simulink model "rx2"  (R2022b)
settings: Solver=FixedStepDiscrete  StartTime=0.0  StopTime=3.3E6  FixedStep=1  RelTol=1e-3  EnableMultiTasking=on
model workspace (MAT data in the model file):
  mwTaskManagerKernelLatency = 0
undefined symbols (not defined in the file or in its folder): Add, jsin, magnitude, rom_pilot_conj_tt, Shift
libraries: hdlsllib x3231, whdlutilities x525, simulink x260, whdlmod x112, whdledac x26, dsphdlmathfun2 x24, commchan3 x1
(part 2 of 59)

== system rx2/process divide/transport_block3 ==
  data_in : Inport
  data_ctrl : Inport  Port=2  OutDataTypeStr=Bus: samplecontrol
  Bus Creator : BusCreator  Inputs=14
  Compare To Constant : hdlsllib/Logic and Bit Operations/Compare To Constant  relop===  const=1  OutDataTypeStr=boolean
  Compare To Constant1 : hdlsllib/Logic and Bit Operations/Compare To Constant  relop===  const=2  OutDataTypeStr=boolean
  Compare To Constant10 : hdlsllib/Logic and Bit Operations/Compare To Constant  relop===  const=11  OutDataTypeStr=boolean
  Compare To Constant11 : hdlsllib/Logic and Bit Operations/Compare To Constant  relop===  const=12  OutDataTypeStr=boolean
  Compare To Constant12 : hdlsllib/Logic and Bit Operations/Compare To Constant  relop===  const=13  OutDataTypeStr=boolean
  Compare To Constant13 : hdlsllib/Logic and Bit Operations/Compare To Constant  relop===  const=14  OutDataTypeStr=boolean
  Compare To Constant2 : hdlsllib/Logic and Bit Operations/Compare To Constant  relop===  const=3  OutDataTypeStr=boolean
  Compare To Constant3 : hdlsllib/Logic and Bit Operations/Compare To Constant  relop===  const=4  OutDataTypeStr=boolean
  Compare To Constant4 : hdlsllib/Logic and Bit Operations/Compare To Constant  relop===  const=5  OutDataTypeStr=boolean
  Compare To Constant5 : hdlsllib/Logic and Bit Operations/Compare To Constant  relop===  const=6  OutDataTypeStr=boolean
  Compare To Constant6 : hdlsllib/Logic and Bit Operations/Compare To Constant  relop===  const=7  OutDataTypeStr=boolean
  Compare To Constant7 : hdlsllib/Logic and Bit Operations/Compare To Constant  relop===  const=8  OutDataTypeStr=boolean
  Compare To Constant8 : hdlsllib/Logic and Bit Operations/Compare To Constant  relop===  const=9  OutDataTypeStr=boolean
  Compare To Constant9 : hdlsllib/Logic and Bit Operations/Compare To Constant  relop===  const=10  OutDataTypeStr=boolean
  Constant : Constant  Value=0  OutDataTypeStr=uint8
  Delay : Delay  DelayLength=1  InitialCondition=0
  Delay1 : Delay  DelayLength=1  InitialCondition=0
  HDL Counter : hdlsllib/Sources/HDL Counter  CountType=Count limited  CountInit=1  CountStep=1  CountMax=14  CountFromType=Initial value  CountFrom=1  CountResetPort=off  CountLoadPort=off  CountEnbPort=on  CountDirPort=off  CountHitOutputPort=off  CountDataType=Unsigned  CountWordLen=8  CountFracLen=0  CountSampTime=1
  Logical Operator : Logic  AllPortsSameDT=off  OutDataTypeStr=boolean
  Mux : Mux  Inputs=14
  Sample Control Bus Selector : whdlutilities/Sample Control Bus Selector  OutputSignals=start,end,valid
  Subsystem1 : Subsystem
  Subsystem10 : Subsystem
  Subsystem11 : Subsystem
  Subsystem12 : Subsystem
  Subsystem13 : Subsystem
  Subsystem14 : Subsystem
  Subsystem2 : Subsystem
  Subsystem3 : Subsystem
  Subsystem4 : Subsystem
  Subsystem5 : Subsystem
  Subsystem6 : Subsystem
  Subsystem7 : Subsystem
  Subsystem8 : Subsystem
  Subsystem9 : Subsystem
  Switch : Switch  Criteria=u2 ~= 0  SaturateOnIntegerOverflow=off  InputSameDT=off
  data_out : Outport  VectorParamsAs1DForOutWhenUnconnected=off
  valid_out : Outport  Port=2  OutDataTypeStr=Bus: RX_BUSOFDM1  VectorParamsAs1DForOutWhenUnconnected=off
  wires:
  data_in/1 -> Delay/1
  HDL Counter/1 -> Switch/1
  Compare To Constant/1 -> Subsystem1/2(select_valid)
  Compare To Constant1/1 -> Subsystem2/2(select_valid)
  Compare To Constant2/1 -> Subsystem3/2(select_valid)
  Compare To Constant3/1 -> Subsystem4/2(select_valid)
  Compare To Constant4/1 -> Subsystem5/2(select_valid)
  Compare To Constant5/1 -> Subsystem6/2(select_valid)
  Compare To Constant6/1 -> Subsystem7/2(select_valid)
  Compare To Constant7/1 -> Subsystem8/2(select_valid)
  Compare To Constant12/1 -> Subsystem13/2(select_valid)
  Compare To Constant11/1 -> Subsystem12/2(select_valid)
  Compare To Constant10/1 -> Subsystem11/2(select_valid)
  Compare To Constant9/1 -> Subsystem10/2(select_valid)
  Compare To Constant8/1 -> Subsystem9/2(select_valid)
  Delay1/1 -> Compare To Constant13/1, Compare To Constant12/1, Compare To Constant11/1, Compare To Constant10/1, Compare To Constant9/1, Compare To Constant8/1, Compare To Constant7/1, Compare To Constant6/1, Compare To Constant5/1, Compare To Constant4/1, Compare To Constant3/1, Compare To Constant2/1, Compare To Constant1/1, Compare To Constant/1
  Delay/1 -> Subsystem2/1(data_in), Subsystem3/1(data_in), Subsystem4/1(data_in), Subsystem5/1(data_in), Subsystem6/1(data_in), Subsystem7/1(data_in), Subsystem8/1(data_in), Subsystem9/1(data_in), Subsystem10/1(data_in), Subsystem11/1(data_in), Subsystem12/1(data_in), Subsystem14/1(data_in), Subsystem13/1(data_in), Subsystem1/1(data_in)
  Compare To Constant13/1 -> Subsystem14/2(select_valid)
  data_ctrl/1 -> Sample Control Bus Selector/1
  Sample Control Bus Selector/3 -> Logical Operator/2, Switch/2
  Switch/1 -> Delay1/1
  Constant/1 -> Switch/3
  Subsystem1/1(data_out) -> Mux/1
  Subsystem2/1(data_out) -> Mux/2
  Subsystem3/1(data_out) -> Mux/3
  Subsystem4/1(data_out) -> Mux/4
  Subsystem5/1(data_out) -> Mux/5
  Subsystem6/1(data_out) -> Mux/6
  Subsystem7/1(data_out) -> Mux/7
  Subsystem8/1(data_out) -> Mux/8
  Subsystem9/1(data_out) -> Mux/9
  Subsystem10/1(data_out) -> Mux/10
  Subsystem11/1(data_out) -> Mux/11
  Subsystem12/1(data_out) -> Mux/12
  Subsystem13/1(data_out) -> Mux/13
  Subsystem14/1(data_out) -> Mux/14
  Subsystem1/2(ctrl_out) -> Bus Creator/1
  Subsystem2/2(ctrl_out) -> Bus Creator/2
  Subsystem3/2(ctrl_out) -> Bus Creator/3
  Subsystem4/2(ctrl_out) -> Bus Creator/4
  Subsystem5/2(ctrl_out) -> Bus Creator/5
  Subsystem6/2(ctrl_out) -> Bus Creator/6
  Subsystem7/2(ctrl_out) -> Bus Creator/7
  Subsystem8/2(ctrl_out) -> Bus Creator/8
  Subsystem9/2(ctrl_out) -> Bus Creator/9
  Subsystem10/2(ctrl_out) -> Bus Creator/10
  Subsystem11/2(ctrl_out) -> Bus Creator/11
  Subsystem12/2(ctrl_out) -> Bus Creator/12
  Subsystem13/2(ctrl_out) -> Bus Creator/13
  Subsystem14/2(ctrl_out) -> Bus Creator/14
  Bus Creator/1 -> valid_out/1
  Mux/1 -> data_out/1
  Sample Control Bus Selector/2 -> Logical Operator/1
  Logical Operator/1 -> HDL Counter/1

== system rx2/process divide/transport_block4 ==
  data_in : Inport
  data_ctrl : Inport  Port=2  OutDataTypeStr=Bus: samplecontrol
  Bus Creator : BusCreator  Inputs=14
  Compare To Constant : hdlsllib/Logic and Bit Operations/Compare To Constant  relop===  const=1  OutDataTypeStr=boolean
  Compare To Constant1 : hdlsllib/Logic and Bit Operations/Compare To Constant  relop===  const=2  OutDataTypeStr=boolean
  Compare To Constant10 : hdlsllib/Logic and Bit Operations/Compare To Constant  relop===  const=11  OutDataTypeStr=boolean
  Compare To Constant11 : hdlsllib/Logic and Bit Operations/Compare To Constant  relop===  const=12  OutDataTypeStr=boolean
  Compare To Constant12 : hdlsllib/Logic and Bit Operations/Compare To Constant  relop===  const=13  OutDataTypeStr=boolean
  Compare To Constant13 : hdlsllib/Logic and Bit Operations/Compare To Constant  relop===  const=14  OutDataTypeStr=boolean
  Compare To Constant2 : hdlsllib/Logic and Bit Operations/Compare To Constant  relop===  const=3  OutDataTypeStr=boolean
  Compare To Constant3 : hdlsllib/Logic and Bit Operations/Compare To Constant  relop===  const=4  OutDataTypeStr=boolean
  Compare To Constant4 : hdlsllib/Logic and Bit Operations/Compare To Constant  relop===  const=5  OutDataTypeStr=boolean
  Compare To Constant5 : hdlsllib/Logic and Bit Operations/Compare To Constant  relop===  const=6  OutDataTypeStr=boolean
  Compare To Constant6 : hdlsllib/Logic and Bit Operations/Compare To Constant  relop===  const=7  OutDataTypeStr=boolean
  Compare To Constant7 : hdlsllib/Logic and Bit Operations/Compare To Constant  relop===  const=8  OutDataTypeStr=boolean
  Compare To Constant8 : hdlsllib/Logic and Bit Operations/Compare To Constant  relop===  const=9  OutDataTypeStr=boolean
  Compare To Constant9 : hdlsllib/Logic and Bit Operations/Compare To Constant  relop===  const=10  OutDataTypeStr=boolean
  Constant : Constant  Value=0  OutDataTypeStr=uint8
  Delay : Delay  DelayLength=1  InitialCondition=0
  Delay1 : Delay  DelayLength=1  InitialCondition=0
  HDL Counter : hdlsllib/Sources/HDL Counter  CountType=Count limited  CountInit=1  CountStep=1  CountMax=14  CountFromType=Initial value  CountFrom=1  CountResetPort=off  CountLoadPort=off  CountEnbPort=on  CountDirPort=off  CountHitOutputPort=off  CountDataType=Unsigned  CountWordLen=8  CountFracLen=0  CountSampTime=1
  Logical Operator : Logic  AllPortsSameDT=off  OutDataTypeStr=boolean
  Mux : Mux  Inputs=14
  Sample Control Bus Selector : whdlutilities/Sample Control Bus Selector  OutputSignals=start,end,valid
  Subsystem1 : Subsystem
  Subsystem10 : Subsystem
  Subsystem11 : Subsystem
  Subsystem12 : Subsystem
  Subsystem13 : Subsystem
  Subsystem14 : Subsystem
  Subsystem2 : Subsystem
  Subsystem3 : Subsystem
  Subsystem4 : Subsystem
  Subsystem5 : Subsystem
  Subsystem6 : Subsystem
  Subsystem7 : Subsystem
  Subsystem8 : Subsystem
  Subsystem9 : Subsystem
  Switch : Switch  Criteria=u2 ~= 0  SaturateOnIntegerOverflow=off  InputSameDT=off
  data_out : Outport  VectorParamsAs1DForOutWhenUnconnected=off
  valid_out : Outport  Port=2  OutDataTypeStr=Bus: RX_BUSOFDM1  VectorParamsAs1DForOutWhenUnconnected=off
  wires:
  Logical Operator/1 -> HDL Counter/1
  Sample Control Bus Selector/2 -> Logical Operator/1
  Mux/1 -> data_out/1
  Bus Creator/1 -> valid_out/1
  Subsystem14/2(ctrl_out) -> Bus Creator/14
  Subsystem13/2(ctrl_out) -> Bus Creator/13
  Subsystem12/2(ctrl_out) -> Bus Creator/12
  Subsystem11/2(ctrl_out) -> Bus Creator/11
  Subsystem10/2(ctrl_out) -> Bus Creator/10
  Subsystem9/2(ctrl_out) -> Bus Creator/9
  Subsystem8/2(ctrl_out) -> Bus Creator/8
  Subsystem7/2(ctrl_out) -> Bus Creator/7
  Subsystem6/2(ctrl_out) -> Bus Creator/6
  Subsystem5/2(ctrl_out) -> Bus Creator/5
  Subsystem4/2(ctrl_out) -> Bus Creator/4
  Subsystem3/2(ctrl_out) -> Bus Creator/3
  Subsystem2/2(ctrl_out) -> Bus Creator/2
  Subsystem1/2(ctrl_out) -> Bus Creator/1
  Subsystem14/1(data_out) -> Mux/14
  Subsystem13/1(data_out) -> Mux/13
  Subsystem12/1(data_out) -> Mux/12
  Subsystem11/1(data_out) -> Mux/11
  Subsystem10/1(data_out) -> Mux/10
  Subsystem9/1(data_out) -> Mux/9
  Subsystem8/1(data_out) -> Mux/8
  Subsystem7/1(data_out) -> Mux/7
  Subsystem6/1(data_out) -> Mux/6
  Subsystem5/1(data_out) -> Mux/5
  Subsystem4/1(data_out) -> Mux/4
  Subsystem3/1(data_out) -> Mux/3
  Subsystem2/1(data_out) -> Mux/2
  Subsystem1/1(data_out) -> Mux/1
  Constant/1 -> Switch/3
  Switch/1 -> Delay1/1
  Sample Control Bus Selector/3 -> Switch/2, Logical Operator/2
  data_ctrl/1 -> Sample Control Bus Selector/1
  Compare To Constant13/1 -> Subsystem14/2(select_valid)
  Delay/1 -> Subsystem1/1(data_in), Subsystem13/1(data_in), Subsystem14/1(data_in), Subsystem12/1(data_in), Subsystem11/1(data_in), Subsystem10/1(data_in), Subsystem9/1(data_in), Subsystem8/1(data_in), Subsystem7/1(data_in), Subsystem6/1(data_in), Subsystem5/1(data_in), Subsystem4/1(data_in), Subsystem3/1(data_in), Subsystem2/1(data_in)
  Delay1/1 -> Compare To Constant/1, Compare To Constant1/1, Compare To Constant2/1, Compare To Constant3/1, Compare To Constant4/1, Compare To Constant5/1, Compare To Constant6/1, Compare To Constant7/1, Compare To Constant8/1, Compare To Constant9/1, Compare To Constant10/1, Compare To Constant11/1, Compare To Constant12/1, Compare To Constant13/1
  Compare To Constant8/1 -> Subsystem9/2(select_valid)
  Compare To Constant9/1 -> Subsystem10/2(select_valid)
  Compare To Constant10/1 -> Subsystem11/2(select_valid)
  Compare To Constant11/1 -> Subsystem12/2(select_valid)
  Compare To Constant12/1 -> Subsystem13/2(select_valid)
  Compare To Constant7/1 -> Subsystem8/2(select_valid)
  Compare To Constant6/1 -> Subsystem7/2(select_valid)
  Compare To Constant5/1 -> Subsystem6/2(select_valid)
  Compare To Constant4/1 -> Subsystem5/2(select_valid)
  Compare To Constant3/1 -> Subsystem4/2(select_valid)
  Compare To Constant2/1 -> Subsystem3/2(select_valid)
  Compare To Constant1/1 -> Subsystem2/2(select_valid)
  Compare To Constant/1 -> Subsystem1/2(select_valid)
  HDL Counter/1 -> Switch/1
  data_in/1 -> Delay/1

== system rx2/process divide/transport_block5 ==
  data_in : Inport
  data_ctrl : Inport  Port=2  OutDataTypeStr=Bus: samplecontrol
  Bus Creator : BusCreator  Inputs=14
  Compare To Constant : hdlsllib/Logic and Bit Operations/Compare To Constant  relop===  const=1  OutDataTypeStr=boolean
  Compare To Constant1 : hdlsllib/Logic and Bit Operations/Compare To Constant  relop===  const=2  OutDataTypeStr=boolean
  Compare To Constant10 : hdlsllib/Logic and Bit Operations/Compare To Constant  relop===  const=11  OutDataTypeStr=boolean
  Compare To Constant11 : hdlsllib/Logic and Bit Operations/Compare To Constant  relop===  const=12  OutDataTypeStr=boolean
  Compare To Constant12 : hdlsllib/Logic and Bit Operations/Compare To Constant  relop===  const=13  OutDataTypeStr=boolean
  Compare To Constant13 : hdlsllib/Logic and Bit Operations/Compare To Constant  relop===  const=14  OutDataTypeStr=boolean
  Compare To Constant2 : hdlsllib/Logic and Bit Operations/Compare To Constant  relop===  const=3  OutDataTypeStr=boolean
  Compare To Constant3 : hdlsllib/Logic and Bit Operations/Compare To Constant  relop===  const=4  OutDataTypeStr=boolean
  Compare To Constant4 : hdlsllib/Logic and Bit Operations/Compare To Constant  relop===  const=5  OutDataTypeStr=boolean
  Compare To Constant5 : hdlsllib/Logic and Bit Operations/Compare To Constant  relop===  const=6  OutDataTypeStr=boolean
  Compare To Constant6 : hdlsllib/Logic and Bit Operations/Compare To Constant  relop===  const=7  OutDataTypeStr=boolean
  Compare To Constant7 : hdlsllib/Logic and Bit Operations/Compare To Constant  relop===  const=8  OutDataTypeStr=boolean
  Compare To Constant8 : hdlsllib/Logic and Bit Operations/Compare To Constant  relop===  const=9  OutDataTypeStr=boolean
  Compare To Constant9 : hdlsllib/Logic and Bit Operations/Compare To Constant  relop===  const=10  OutDataTypeStr=boolean
  Constant : Constant  Value=0  OutDataTypeStr=uint8
  Delay : Delay  DelayLength=1  InitialCondition=0
  Delay1 : Delay  DelayLength=1  InitialCondition=0
  HDL Counter : hdlsllib/Sources/HDL Counter  CountType=Count limited  CountInit=1  CountStep=1  CountMax=14  CountFromType=Initial value  CountFrom=1  CountResetPort=off  CountLoadPort=off  CountEnbPort=on  CountDirPort=off  CountHitOutputPort=off  CountDataType=Unsigned  CountWordLen=8  CountFracLen=0  CountSampTime=1
  Logical Operator : Logic  AllPortsSameDT=off  OutDataTypeStr=boolean
  Mux : Mux  Inputs=14
  Sample Control Bus Selector : whdlutilities/Sample Control Bus Selector  OutputSignals=start,end,valid
  Subsystem1 : Subsystem
  Subsystem10 : Subsystem
  Subsystem11 : Subsystem
  Subsystem12 : Subsystem
  Subsystem13 : Subsystem
  Subsystem14 : Subsystem
  Subsystem2 : Subsystem
  Subsystem3 : Subsystem
  Subsystem4 : Subsystem
  Subsystem5 : Subsystem
  Subsystem6 : Subsystem
  Subsystem7 : Subsystem
  Subsystem8 : Subsystem
  Subsystem9 : Subsystem
  Switch : Switch  Criteria=u2 ~= 0  SaturateOnIntegerOverflow=off  InputSameDT=off
  data_out : Outport  VectorParamsAs1DForOutWhenUnconnected=off
  valid_out : Outport  Port=2  OutDataTypeStr=Bus: RX_BUSOFDM1  VectorParamsAs1DForOutWhenUnconnected=off
  wires:
  data_in/1 -> Delay/1
  HDL Counter/1 -> Switch/1
  Compare To Constant/1 -> Subsystem1/2(select_valid)
  Compare To Constant1/1 -> Subsystem2/2(select_valid)
  Compare To Constant2/1 -> Subsystem3/2(select_valid)
  Compare To Constant3/1 -> Subsystem4/2(select_valid)
  Compare To Constant4/1 -> Subsystem5/2(select_valid)
  Compare To Constant5/1 -> Subsystem6/2(select_valid)
  Compare To Constant6/1 -> Subsystem7/2(select_valid)
  Compare To Constant7/1 -> Subsystem8/2(select_valid)
  Compare To Constant12/1 -> Subsystem13/2(select_valid)
  Compare To Constant11/1 -> Subsystem12/2(select_valid)
  Compare To Constant10/1 -> Subsystem11/2(select_valid)
  Compare To Constant9/1 -> Subsystem10/2(select_valid)
  Compare To Constant8/1 -> Subsystem9/2(select_valid)
  Delay1/1 -> Compare To Constant13/1, Compare To Constant12/1, Compare To Constant11/1, Compare To Constant10/1, Compare To Constant9/1, Compare To Constant8/1, Compare To Constant7/1, Compare To Constant6/1, Compare To Constant5/1, Compare To Constant4/1, Compare To Constant3/1, Compare To Constant2/1, Compare To Constant1/1, Compare To Constant/1
  Delay/1 -> Subsystem2/1(data_in), Subsystem3/1(data_in), Subsystem4/1(data_in), Subsystem5/1(data_in), Subsystem6/1(data_in), Subsystem7/1(data_in), Subsystem8/1(data_in), Subsystem9/1(data_in), Subsystem10/1(data_in), Subsystem11/1(data_in), Subsystem12/1(data_in), Subsystem14/1(data_in), Subsystem13/1(data_in), Subsystem1/1(data_in)
  Compare To Constant13/1 -> Subsystem14/2(select_valid)
  data_ctrl/1 -> Sample Control Bus Selector/1
  Sample Control Bus Selector/3 -> Logical Operator/2, Switch/2
  Switch/1 -> Delay1/1
  Constant/1 -> Switch/3
  Subsystem1/1(data_out) -> Mux/1
  Subsystem2/1(data_out) -> Mux/2
  Subsystem3/1(data_out) -> Mux/3
  Subsystem4/1(data_out) -> Mux/4
  Subsystem5/1(data_out) -> Mux/5
  Subsystem6/1(data_out) -> Mux/6
  Subsystem7/1(data_out) -> Mux/7
  Subsystem8/1(data_out) -> Mux/8
  Subsystem9/1(data_out) -> Mux/9
  Subsystem10/1(data_out) -> Mux/10
  Subsystem11/1(data_out) -> Mux/11
  Subsystem12/1(data_out) -> Mux/12
  Subsystem13/1(data_out) -> Mux/13
  Subsystem14/1(data_out) -> Mux/14
  Subsystem1/2(ctrl_out) -> Bus Creator/1
  Subsystem2/2(ctrl_out) -> Bus Creator/2
  Subsystem3/2(ctrl_out) -> Bus Creator/3
  Subsystem4/2(ctrl_out) -> Bus Creator/4
  Subsystem5/2(ctrl_out) -> Bus Creator/5
  Subsystem6/2(ctrl_out) -> Bus Creator/6
  Subsystem7/2(ctrl_out) -> Bus Creator/7
  Subsystem8/2(ctrl_out) -> Bus Creator/8
  Subsystem9/2(ctrl_out) -> Bus Creator/9
  Subsystem10/2(ctrl_out) -> Bus Creator/10
  Subsystem11/2(ctrl_out) -> Bus Creator/11
  Subsystem12/2(ctrl_out) -> Bus Creator/12
  Subsystem13/2(ctrl_out) -> Bus Creator/13
  Subsystem14/2(ctrl_out) -> Bus Creator/14
  Bus Creator/1 -> valid_out/1
  Mux/1 -> data_out/1
  Sample Control Bus Selector/2 -> Logical Operator/1
  Logical Operator/1 -> HDL Counter/1

== system rx2/process divide/transport_block6 ==
  data_in : Inport
  data_ctrl : Inport  Port=2  OutDataTypeStr=Bus: samplecontrol
  Bus Creator : BusCreator  Inputs=14
  Compare To Constant : hdlsllib/Logic and Bit Operations/Compare To Constant  relop===  const=1  OutDataTypeStr=boolean
  Compare To Constant1 : hdlsllib/Logic and Bit Operations/Compare To Constant  relop===  const=2  OutDataTypeStr=boolean
  Compare To Constant10 : hdlsllib/Logic and Bit Operations/Compare To Constant  relop===  const=11  OutDataTypeStr=boolean
  Compare To Constant11 : hdlsllib/Logic and Bit Operations/Compare To Constant  relop===  const=12  OutDataTypeStr=boolean
  Compare To Constant12 : hdlsllib/Logic and Bit Operations/Compare To Constant  relop===  const=13  OutDataTypeStr=boolean
  Compare To Constant13 : hdlsllib/Logic and Bit Operations/Compare To Constant  relop===  const=14  OutDataTypeStr=boolean
  Compare To Constant2 : hdlsllib/Logic and Bit Operations/Compare To Constant  relop===  const=3  OutDataTypeStr=boolean
  Compare To Constant3 : hdlsllib/Logic and Bit Operations/Compare To Constant  relop===  const=4  OutDataTypeStr=boolean
  Compare To Constant4 : hdlsllib/Logic and Bit Operations/Compare To Constant  relop===  const=5  OutDataTypeStr=boolean
  Compare To Constant5 : hdlsllib/Logic and Bit Operations/Compare To Constant  relop===  const=6  OutDataTypeStr=boolean
  Compare To Constant6 : hdlsllib/Logic and Bit Operations/Compare To Constant  relop===  const=7  OutDataTypeStr=boolean
  Compare To Constant7 : hdlsllib/Logic and Bit Operations/Compare To Constant  relop===  const=8  OutDataTypeStr=boolean
  Compare To Constant8 : hdlsllib/Logic and Bit Operations/Compare To Constant  relop===  const=9  OutDataTypeStr=boolean
  Compare To Constant9 : hdlsllib/Logic and Bit Operations/Compare To Constant  relop===  const=10  OutDataTypeStr=boolean
  Constant : Constant  Value=0  OutDataTypeStr=uint8
  Delay : Delay  DelayLength=1  InitialCondition=0
  Delay1 : Delay  DelayLength=1  InitialCondition=0
  HDL Counter : hdlsllib/Sources/HDL Counter  CountType=Count limited  CountInit=1  CountStep=1  CountMax=14  CountFromType=Initial value  CountFrom=1  CountResetPort=off  CountLoadPort=off  CountEnbPort=on  CountDirPort=off  CountHitOutputPort=off  CountDataType=Unsigned  CountWordLen=8  CountFracLen=0  CountSampTime=1
  Logical Operator : Logic  AllPortsSameDT=off  OutDataTypeStr=boolean
  Mux : Mux  Inputs=14
  Sample Control Bus Selector : whdlutilities/Sample Control Bus Selector  OutputSignals=start,end,valid
  Subsystem1 : Subsystem
  Subsystem10 : Subsystem
  Subsystem11 : Subsystem
  Subsystem12 : Subsystem
  Subsystem13 : Subsystem
  Subsystem14 : Subsystem
  Subsystem2 : Subsystem
  Subsystem3 : Subsystem
  Subsystem4 : Subsystem
  Subsystem5 : Subsystem
  Subsystem6 : Subsystem
  Subsystem7 : Subsystem
  Subsystem8 : Subsystem
  Subsystem9 : Subsystem
  Switch : Switch  Criteria=u2 ~= 0  SaturateOnIntegerOverflow=off  InputSameDT=off
  data_out : Outport  VectorParamsAs1DForOutWhenUnconnected=off
  valid_out : Outport  Port=2  OutDataTypeStr=Bus: RX_BUSOFDM1  VectorParamsAs1DForOutWhenUnconnected=off
  wires:
  Logical Operator/1 -> HDL Counter/1
  Sample Control Bus Selector/2 -> Logical Operator/1
  Mux/1 -> data_out/1
  Bus Creator/1 -> valid_out/1
  Subsystem14/2(ctrl_out) -> Bus Creator/14
  Subsystem13/2(ctrl_out) -> Bus Creator/13
  Subsystem12/2(ctrl_out) -> Bus Creator/12
  Subsystem11/2(ctrl_out) -> Bus Creator/11
  Subsystem10/2(ctrl_out) -> Bus Creator/10
  Subsystem9/2(ctrl_out) -> Bus Creator/9
  Subsystem8/2(ctrl_out) -> Bus Creator/8
  Subsystem7/2(ctrl_out) -> Bus Creator/7
  Subsystem6/2(ctrl_out) -> Bus Creator/6
  Subsystem5/2(ctrl_out) -> Bus Creator/5
  Subsystem4/2(ctrl_out) -> Bus Creator/4
  Subsystem3/2(ctrl_out) -> Bus Creator/3
  Subsystem2/2(ctrl_out) -> Bus Creator/2
  Subsystem1/2(ctrl_out) -> Bus Creator/1
  Subsystem14/1(data_out) -> Mux/14
  Subsystem13/1(data_out) -> Mux/13
  Subsystem12/1(data_out) -> Mux/12
  Subsystem11/1(data_out) -> Mux/11
  Subsystem10/1(data_out) -> Mux/10
  Subsystem9/1(data_out) -> Mux/9
  Subsystem8/1(data_out) -> Mux/8
  Subsystem7/1(data_out) -> Mux/7
  Subsystem6/1(data_out) -> Mux/6
  Subsystem5/1(data_out) -> Mux/5
  Subsystem4/1(data_out) -> Mux/4
  Subsystem3/1(data_out) -> Mux/3
  Subsystem2/1(data_out) -> Mux/2
  Subsystem1/1(data_out) -> Mux/1
  Constant/1 -> Switch/3
  Switch/1 -> Delay1/1
  Sample Control Bus Selector/3 -> Switch/2, Logical Operator/2
  data_ctrl/1 -> Sample Control Bus Selector/1
  Compare To Constant13/1 -> Subsystem14/2(select_valid)
  Delay/1 -> Subsystem1/1(data_in), Subsystem13/1(data_in), Subsystem14/1(data_in), Subsystem12/1(data_in), Subsystem11/1(data_in), Subsystem10/1(data_in), Subsystem9/1(data_in), Subsystem8/1(data_in), Subsystem7/1(data_in), Subsystem6/1(data_in), Subsystem5/1(data_in), Subsystem4/1(data_in), Subsystem3/1(data_in), Subsystem2/1(data_in)
  Delay1/1 -> Compare To Constant/1, Compare To Constant1/1, Compare To Constant2/1, Compare To Constant3/1, Compare To Constant4/1, Compare To Constant5/1, Compare To Constant6/1, Compare To Constant7/1, Compare To Constant8/1, Compare To Constant9/1, Compare To Constant10/1, Compare To Constant11/1, Compare To Constant12/1, Compare To Constant13/1
  Compare To Constant8/1 -> Subsystem9/2(select_valid)
  Compare To Constant9/1 -> Subsystem10/2(select_valid)
  Compare To Constant10/1 -> Subsystem11/2(select_valid)
  Compare To Constant11/1 -> Subsystem12/2(select_valid)
  Compare To Constant12/1 -> Subsystem13/2(select_valid)
  Compare To Constant7/1 -> Subsystem8/2(select_valid)
  Compare To Constant6/1 -> Subsystem7/2(select_valid)
  Compare To Constant5/1 -> Subsystem6/2(select_valid)
  Compare To Constant4/1 -> Subsystem5/2(select_valid)
  Compare To Constant3/1 -> Subsystem4/2(select_valid)
  Compare To Constant2/1 -> Subsystem3/2(select_valid)
  Compare To Constant1/1 -> Subsystem2/2(select_valid)
  Compare To Constant/1 -> Subsystem1/2(select_valid)
  HDL Counter/1 -> Switch/1
  data_in/1 -> Delay/1

== system rx2/process divide/transport_block7 ==
  data_in : Inport
  data_ctrl : Inport  Port=2  OutDataTypeStr=Bus: samplecontrol
  Bus Creator : BusCreator  Inputs=14
  Compare To Constant : hdlsllib/Logic and Bit Operations/Compare To Constant  relop===  const=1  OutDataTypeStr=boolean
  Compare To Constant1 : hdlsllib/Logic and Bit Operations/Compare To Constant  relop===  const=2  OutDataTypeStr=boolean
  Compare To Constant10 : hdlsllib/Logic and Bit Operations/Compare To Constant  relop===  const=11  OutDataTypeStr=boolean
  Compare To Constant11 : hdlsllib/Logic and Bit Operations/Compare To Constant  relop===  const=12  OutDataTypeStr=boolean
  Compare To Constant12 : hdlsllib/Logic and Bit Operations/Compare To Constant  relop===  const=13  OutDataTypeStr=boolean
  Compare To Constant13 : hdlsllib/Logic and Bit Operations/Compare To Constant  relop===  const=14  OutDataTypeStr=boolean
  Compare To Constant2 : hdlsllib/Logic and Bit Operations/Compare To Constant  relop===  const=3  OutDataTypeStr=boolean
  Compare To Constant3 : hdlsllib/Logic and Bit Operations/Compare To Constant  relop===  const=4  OutDataTypeStr=boolean
  Compare To Constant4 : hdlsllib/Logic and Bit Operations/Compare To Constant  relop===  const=5  OutDataTypeStr=boolean
  Compare To Constant5 : hdlsllib/Logic and Bit Operations/Compare To Constant  relop===  const=6  OutDataTypeStr=boolean
  Compare To Constant6 : hdlsllib/Logic and Bit Operations/Compare To Constant  relop===  const=7  OutDataTypeStr=boolean
  Compare To Constant7 : hdlsllib/Logic and Bit Operations/Compare To Constant  relop===  const=8  OutDataTypeStr=boolean
  Compare To Constant8 : hdlsllib/Logic and Bit Operations/Compare To Constant  relop===  const=9  OutDataTypeStr=boolean
  Compare To Constant9 : hdlsllib/Logic and Bit Operations/Compare To Constant  relop===  const=10  OutDataTypeStr=boolean
  Constant : Constant  Value=0  OutDataTypeStr=uint8
  Delay : Delay  DelayLength=1  InitialCondition=0
  Delay1 : Delay  DelayLength=1  InitialCondition=0
  HDL Counter : hdlsllib/Sources/HDL Counter  CountType=Count limited  CountInit=1  CountStep=1  CountMax=14  CountFromType=Initial value  CountFrom=1  CountResetPort=off  CountLoadPort=off  CountEnbPort=on  CountDirPort=off  CountHitOutputPort=off  CountDataType=Unsigned  CountWordLen=8  CountFracLen=0  CountSampTime=1
  Logical Operator : Logic  AllPortsSameDT=off  OutDataTypeStr=boolean
  Mux : Mux  Inputs=14
  Sample Control Bus Selector : whdlutilities/Sample Control Bus Selector  OutputSignals=start,end,valid
  Subsystem1 : Subsystem
  Subsystem10 : Subsystem
  Subsystem11 : Subsystem
  Subsystem12 : Subsystem
  Subsystem13 : Subsystem
  Subsystem14 : Subsystem
  Subsystem2 : Subsystem
  Subsystem3 : Subsystem
  Subsystem4 : Subsystem
  Subsystem5 : Subsystem
  Subsystem6 : Subsystem
  Subsystem7 : Subsystem
  Subsystem8 : Subsystem
  Subsystem9 : Subsystem
  Switch : Switch  Criteria=u2 ~= 0  SaturateOnIntegerOverflow=off  InputSameDT=off
  data_out : Outport  VectorParamsAs1DForOutWhenUnconnected=off
  valid_out : Outport  Port=2  OutDataTypeStr=Bus: RX_BUSOFDM1  VectorParamsAs1DForOutWhenUnconnected=off
  wires:
  data_in/1 -> Delay/1
  HDL Counter/1 -> Switch/1
  Compare To Constant/1 -> Subsystem1/2(select_valid)
  Compare To Constant1/1 -> Subsystem2/2(select_valid)
  Compare To Constant2/1 -> Subsystem3/2(select_valid)
  Compare To Constant3/1 -> Subsystem4/2(select_valid)
  Compare To Constant4/1 -> Subsystem5/2(select_valid)
  Compare To Constant5/1 -> Subsystem6/2(select_valid)
  Compare To Constant6/1 -> Subsystem7/2(select_valid)
  Compare To Constant7/1 -> Subsystem8/2(select_valid)
  Compare To Constant12/1 -> Subsystem13/2(select_valid)
  Compare To Constant11/1 -> Subsystem12/2(select_valid)
  Compare To Constant10/1 -> Subsystem11/2(select_valid)
  Compare To Constant9/1 -> Subsystem10/2(select_valid)
  Compare To Constant8/1 -> Subsystem9/2(select_valid)
  Delay1/1 -> Compare To Constant13/1, Compare To Constant12/1, Compare To Constant11/1, Compare To Constant10/1, Compare To Constant9/1, Compare To Constant8/1, Compare To Constant7/1, Compare To Constant6/1, Compare To Constant5/1, Compare To Constant4/1, Compare To Constant3/1, Compare To Constant2/1, Compare To Constant1/1, Compare To Constant/1
  Delay/1 -> Subsystem2/1(data_in), Subsystem3/1(data_in), Subsystem4/1(data_in), Subsystem5/1(data_in), Subsystem6/1(data_in), Subsystem7/1(data_in), Subsystem8/1(data_in), Subsystem9/1(data_in), Subsystem10/1(data_in), Subsystem11/1(data_in), Subsystem12/1(data_in), Subsystem14/1(data_in), Subsystem13/1(data_in), Subsystem1/1(data_in)
  Compare To Constant13/1 -> Subsystem14/2(select_valid)
  data_ctrl/1 -> Sample Control Bus Selector/1
  Sample Control Bus Selector/3 -> Logical Operator/2, Switch/2
  Switch/1 -> Delay1/1
  Constant/1 -> Switch/3
  Subsystem1/1(data_out) -> Mux/1
  Subsystem2/1(data_out) -> Mux/2
  Subsystem3/1(data_out) -> Mux/3
  Subsystem4/1(data_out) -> Mux/4
  Subsystem5/1(data_out) -> Mux/5
  Subsystem6/1(data_out) -> Mux/6
  Subsystem7/1(data_out) -> Mux/7
  Subsystem8/1(data_out) -> Mux/8
  Subsystem9/1(data_out) -> Mux/9
  Subsystem10/1(data_out) -> Mux/10
  Subsystem11/1(data_out) -> Mux/11
  Subsystem12/1(data_out) -> Mux/12
  Subsystem13/1(data_out) -> Mux/13
  Subsystem14/1(data_out) -> Mux/14
  Subsystem1/2(ctrl_out) -> Bus Creator/1
  Subsystem2/2(ctrl_out) -> Bus Creator/2
  Subsystem3/2(ctrl_out) -> Bus Creator/3
  Subsystem4/2(ctrl_out) -> Bus Creator/4
  Subsystem5/2(ctrl_out) -> Bus Creator/5
  Subsystem6/2(ctrl_out) -> Bus Creator/6
  Subsystem7/2(ctrl_out) -> Bus Creator/7
  Subsystem8/2(ctrl_out) -> Bus Creator/8
  Subsystem9/2(ctrl_out) -> Bus Creator/9
  Subsystem10/2(ctrl_out) -> Bus Creator/10
  Subsystem11/2(ctrl_out) -> Bus Creator/11
  Subsystem12/2(ctrl_out) -> Bus Creator/12
  Subsystem13/2(ctrl_out) -> Bus Creator/13
  Subsystem14/2(ctrl_out) -> Bus Creator/14
  Bus Creator/1 -> valid_out/1
  Mux/1 -> data_out/1
  Sample Control Bus Selector/2 -> Logical Operator/1
  Logical Operator/1 -> HDL Counter/1

== system rx2/process divide/transport_block8 ==
  data_in : Inport
  data_ctrl : Inport  Port=2  OutDataTypeStr=Bus: samplecontrol
  Bus Creator : BusCreator  Inputs=14
  Compare To Constant : hdlsllib/Logic and Bit Operations/Compare To Constant  relop===  const=1  OutDataTypeStr=boolean
  Compare To Constant1 : hdlsllib/Logic and Bit Operations/Compare To Constant  relop===  const=2  OutDataTypeStr=boolean
  Compare To Constant10 : hdlsllib/Logic and Bit Operations/Compare To Constant  relop===  const=11  OutDataTypeStr=boolean
  Compare To Constant11 : hdlsllib/Logic and Bit Operations/Compare To Constant  relop===  const=12  OutDataTypeStr=boolean
  Compare To Constant12 : hdlsllib/Logic and Bit Operations/Compare To Constant  relop===  const=13  OutDataTypeStr=boolean
  Compare To Constant13 : hdlsllib/Logic and Bit Operations/Compare To Constant  relop===  const=14  OutDataTypeStr=boolean
  Compare To Constant2 : hdlsllib/Logic and Bit Operations/Compare To Constant  relop===  const=3  OutDataTypeStr=boolean
  Compare To Constant3 : hdlsllib/Logic and Bit Operations/Compare To Constant  relop===  const=4  OutDataTypeStr=boolean
  Compare To Constant4 : hdlsllib/Logic and Bit Operations/Compare To Constant  relop===  const=5  OutDataTypeStr=boolean
  Compare To Constant5 : hdlsllib/Logic and Bit Operations/Compare To Constant  relop===  const=6  OutDataTypeStr=boolean
  Compare To Constant6 : hdlsllib/Logic and Bit Operations/Compare To Constant  relop===  const=7  OutDataTypeStr=boolean
  Compare To Constant7 : hdlsllib/Logic and Bit Operations/Compare To Constant  relop===  const=8  OutDataTypeStr=boolean
  Compare To Constant8 : hdlsllib/Logic and Bit Operations/Compare To Constant  relop===  const=9  OutDataTypeStr=boolean
  Compare To Constant9 : hdlsllib/Logic and Bit Operations/Compare To Constant  relop===  const=10  OutDataTypeStr=boolean
  Constant : Constant  Value=0  OutDataTypeStr=uint8
  Delay : Delay  DelayLength=1  InitialCondition=0
  Delay1 : Delay  DelayLength=1  InitialCondition=0
  HDL Counter : hdlsllib/Sources/HDL Counter  CountType=Count limited  CountInit=1  CountStep=1  CountMax=14  CountFromType=Initial value  CountFrom=1  CountResetPort=off  CountLoadPort=off  CountEnbPort=on  CountDirPort=off  CountHitOutputPort=off  CountDataType=Unsigned  CountWordLen=8  CountFracLen=0  CountSampTime=1
  Logical Operator : Logic  AllPortsSameDT=off  OutDataTypeStr=boolean
  Mux : Mux  Inputs=14
  Sample Control Bus Selector : whdlutilities/Sample Control Bus Selector  OutputSignals=start,end,valid
  Subsystem1 : Subsystem
  Subsystem10 : Subsystem
  Subsystem11 : Subsystem
  Subsystem12 : Subsystem
  Subsystem13 : Subsystem
  Subsystem14 : Subsystem
  Subsystem2 : Subsystem
  Subsystem3 : Subsystem
  Subsystem4 : Subsystem
  Subsystem5 : Subsystem
  Subsystem6 : Subsystem
  Subsystem7 : Subsystem
  Subsystem8 : Subsystem
  Subsystem9 : Subsystem
  Switch : Switch  Criteria=u2 ~= 0  SaturateOnIntegerOverflow=off  InputSameDT=off
  data_out : Outport  VectorParamsAs1DForOutWhenUnconnected=off
  valid_out : Outport  Port=2  OutDataTypeStr=Bus: RX_BUSOFDM1  VectorParamsAs1DForOutWhenUnconnected=off
  wires:
  Logical Operator/1 -> HDL Counter/1
  Sample Control Bus Selector/2 -> Logical Operator/1
  Mux/1 -> data_out/1
  Bus Creator/1 -> valid_out/1
  Subsystem14/2(ctrl_out) -> Bus Creator/14
  Subsystem13/2(ctrl_out) -> Bus Creator/13
  Subsystem12/2(ctrl_out) -> Bus Creator/12
  Subsystem11/2(ctrl_out) -> Bus Creator/11
  Subsystem10/2(ctrl_out) -> Bus Creator/10
  Subsystem9/2(ctrl_out) -> Bus Creator/9
  Subsystem8/2(ctrl_out) -> Bus Creator/8
  Subsystem7/2(ctrl_out) -> Bus Creator/7
  Subsystem6/2(ctrl_out) -> Bus Creator/6
  Subsystem5/2(ctrl_out) -> Bus Creator/5
  Subsystem4/2(ctrl_out) -> Bus Creator/4
  Subsystem3/2(ctrl_out) -> Bus Creator/3
  Subsystem2/2(ctrl_out) -> Bus Creator/2
  Subsystem1/2(ctrl_out) -> Bus Creator/1
  Subsystem14/1(data_out) -> Mux/14
  Subsystem13/1(data_out) -> Mux/13
  Subsystem12/1(data_out) -> Mux/12
  Subsystem11/1(data_out) -> Mux/11
  Subsystem10/1(data_out) -> Mux/10
  Subsystem9/1(data_out) -> Mux/9
  Subsystem8/1(data_out) -> Mux/8
  Subsystem7/1(data_out) -> Mux/7
  Subsystem6/1(data_out) -> Mux/6
  Subsystem5/1(data_out) -> Mux/5
  Subsystem4/1(data_out) -> Mux/4
  Subsystem3/1(data_out) -> Mux/3
  Subsystem2/1(data_out) -> Mux/2
  Subsystem1/1(data_out) -> Mux/1
  Constant/1 -> Switch/3
  Switch/1 -> Delay1/1
  Sample Control Bus Selector/3 -> Switch/2, Logical Operator/2
  data_ctrl/1 -> Sample Control Bus Selector/1
  Compare To Constant13/1 -> Subsystem14/2(select_valid)
  Delay/1 -> Subsystem1/1(data_in), Subsystem13/1(data_in), Subsystem14/1(data_in), Subsystem12/1(data_in), Subsystem11/1(data_in), Subsystem10/1(data_in), Subsystem9/1(data_in), Subsystem8/1(data_in), Subsystem7/1(data_in), Subsystem6/1(data_in), Subsystem5/1(data_in), Subsystem4/1(data_in), Subsystem3/1(data_in), Subsystem2/1(data_in)
  Delay1/1 -> Compare To Constant/1, Compare To Constant1/1, Compare To Constant2/1, Compare To Constant3/1, Compare To Constant4/1, Compare To Constant5/1, Compare To Constant6/1, Compare To Constant7/1, Compare To Constant8/1, Compare To Constant9/1, Compare To Constant10/1, Compare To Constant11/1, Compare To Constant12/1, Compare To Constant13/1
  Compare To Constant8/1 -> Subsystem9/2(select_valid)
  Compare To Constant9/1 -> Subsystem10/2(select_valid)
  Compare To Constant10/1 -> Subsystem11/2(select_valid)
  Compare To Constant11/1 -> Subsystem12/2(select_valid)
  Compare To Constant12/1 -> Subsystem13/2(select_valid)
  Compare To Constant7/1 -> Subsystem8/2(select_valid)
  Compare To Constant6/1 -> Subsystem7/2(select_valid)
  Compare To Constant5/1 -> Subsystem6/2(select_valid)
  Compare To Constant4/1 -> Subsystem5/2(select_valid)
  Compare To Constant3/1 -> Subsystem4/2(select_valid)
  Compare To Constant2/1 -> Subsystem3/2(select_valid)
  Compare To Constant1/1 -> Subsystem2/2(select_valid)
  Compare To Constant/1 -> Subsystem1/2(select_valid)
  HDL Counter/1 -> Switch/1
  data_in/1 -> Delay/1

== system rx2/process1/OFDM_DEMOD1 ==
  process : Inport
  process_ctrl : Inport  Port=2  OutDataTypeStr=Bus: BUSOFDM1
  Bus Creator : BusCreator  Inputs=8
  Bus Selector : BusSelector  OutputSignals=signal2 (signal 1).valid,signal2 (signal 2).valid,signal2 (signal 3).valid,signal2 (signal 4).valid,signal2 (signal 5).valid,signal2 (signal 6).valid,signal2 (signal 7).valid,signal2 (signal 8).valid
  Demux : Demux  Outputs=8
  Mux : Mux  Inputs=8
  OFDM_demod1 : Subsystem
  OFDM_demod2 : Subsystem
  OFDM_demod3 : Subsystem
  OFDM_demod4 : Subsystem
  OFDM_demod5 : Subsystem
  OFDM_demod6 : Subsystem
  OFDM_demod7 : Subsystem
  OFDM_demod8 : Subsystem
  rxsig : Outport
  Rcrtl_out : Outport  Port=2  OutDataTypeStr=Bus: BUSOFDM1
  wires:
  process_ctrl/1 -> Bus Selector/1
  process/1 -> Demux/1
  Demux/1 -> OFDM_demod1/1(ofdm_sym)
  Demux/2 -> OFDM_demod2/1(ofdm_sym)
  Bus Selector/2 -> OFDM_demod2/2(valid_in)  "<valid>"
  Demux/3 -> OFDM_demod3/1(ofdm_sym)
  Bus Selector/3 -> OFDM_demod3/2(valid_in)  "<valid>"
  Demux/4 -> OFDM_demod4/1(ofdm_sym)
  Bus Selector/4 -> OFDM_demod4/2(valid_in)  "<valid>"
  Bus Selector/5 -> OFDM_demod5/2(valid_in)  "<valid>"
  Bus Selector/6 -> OFDM_demod6/2(valid_in)  "<valid>"
  Bus Selector/7 -> OFDM_demod8/2(valid_in)  "<valid>"
  Bus Selector/8 -> OFDM_demod7/2(valid_in)  "<valid>"
  Demux/5 -> OFDM_demod5/1(ofdm_sym)
  Demux/6 -> OFDM_demod6/1(ofdm_sym)
  Demux/7 -> OFDM_demod8/1(ofdm_sym)
  Demux/8 -> OFDM_demod7/1(ofdm_sym)
  Bus Selector/1 -> OFDM_demod1/2(valid_in)  "<valid>"
  OFDM_demod5/2(ctrl_out) -> Bus Creator/5  "OFDM_ctrl_bf1_process5"
  OFDM_demod2/1(data_out) -> Mux/2
  OFDM_demod7/2(ctrl_out) -> Bus Creator/8  "OFDM_ctrl_bf1_process8"
  OFDM_demod3/1(data_out) -> Mux/3
  OFDM_demod3/2(ctrl_out) -> Bus Creator/3  "OFDM_ctrl_bf1_process3"
  OFDM_demod8/2(ctrl_out) -> Bus Creator/7  "OFDM_ctrl_bf1_process7"
  OFDM_demod5/1(data_out) -> Mux/5
  OFDM_demod1/1(data_out) -> Mux/1
  OFDM_demod2/2(ctrl_out) -> Bus Creator/2  "OFDM_ctrl_bf1_process2"
  OFDM_demod6/2(ctrl_out) -> Bus Creator/6  "OFDM_ctrl_bf1_process6"
  OFDM_demod8/1(data_out) -> Mux/7
  OFDM_demod6/1(data_out) -> Mux/6
  OFDM_demod4/2(ctrl_out) -> Bus Creator/4  "OFDM_ctrl_bf1_process4"
  OFDM_demod1/2(ctrl_out) -> Bus Creator/1  "OFDM_ctrl_bf1_process1"
  OFDM_demod4/1(data_out) -> Mux/4
  OFDM_demod7/1(data_out) -> Mux/8
  Mux/1 -> rxsig/1
  Bus Creator/1 -> Rcrtl_out/1

== system rx2/process1/decoder ==
  chan_est_tt1 : Inport
  port1_ctrl : Inport  Port=2  OutDataTypeStr=Bus: BUSOFDM1
  rxSig_tt1 : Inport  Port=3
  port2_ctrl : Inport  Port=4  OutDataTypeStr=Bus: BUSOFDM1
  nVar_tt : Inport  Port=5  OutDataTypeStr=fixdt(0,16,12)
  Constant2 : Constant  OutDataTypeStr=boolean
  Constant3 : Constant  Value=72  OutDataTypeStr=uint16
  Delay1 : Delay  InitialCondition=0
  Delay2 : Delay  InitialCondition=0
  Detect Rise Positive : hdlsllib/Logic and Bit Operations/Detect Rise Positive  vinit=0  OutDataTypeStr=boolean
  Detect Rise Positive1 : hdlsllib/Logic and Bit Operations/Detect Rise Positive  vinit=0  OutDataTypeStr=boolean
  MRC : Subsystem
  NR CRC Decoder : whdledac/NR CRC Decoder  CRCType=CRC16  FullCheckSum=on  EnableCRCMaskPort=off  SimulateUsing=Code generation
  NR LDPC Decoder : whdledac/NR LDPC Decoder  Algorithm=Min-sum  ScalingFactor=0.75  Termination=Max  SpecifyInputs=Property  NumIterations=15  MaxNumIterations=30  RateCompatible=off  ParityCheckStatus=off  SimulateUsing=Code generation
  Sample Control Bus Selector1 : whdlutilities/Sample Control Bus Selector  OutputSignals=start,end,valid
  deinterleave : Subsystem  mask{length=1584}
      mask prompts: length "the length of data_in"
      mask DialogControl ParameterGroupVar Prompt: 参数
      mask DialogControl Control2 Prompt: the lantency is (length/2+3)
  p-p : Subsystem
  rate recover : Subsystem
  s-p : Subsystem
  soft demodule : Subsystem  mask{demod_length=1584}
      mask prompts: demod_length "The length of demod"
      mask DialogControl ParameterGroupVar Prompt: 参数
      mask DialogControl Control2 Prompt: Latency=4
  synchronization : Subsystem
  synchronize_valid : Subsystem  mask{valid_length=792}
      mask prompts: valid_length "The length of valid"
      mask DialogControl Control2 Prompt: Latency=2
  data_out : Outport
  valid_out : Outport  Port=2
  wires:
  s-p/2(ctrl_out) -> NR LDPC Decoder/2  "ldpc_in_ctrl"
  p-p/1(data) -> NR CRC Decoder/1  "crc_in"
  p-p/2(ctrl) -> NR CRC Decoder/2  "crc_in_ctrl"
  deinterleave/1(data_out) -> rate recover/1(demod)  "deinterleave_data"
  NR LDPC Decoder/2 -> Sample Control Bus Selector1/1  "ldpc_out_ctrl"
  NR LDPC Decoder/1 -> p-p/1(data_in)  "ldpc_out"
  rate recover/1(rate_recover) -> s-p/1(data_in)  "rm_out"
  Detect Rise Positive/1 -> rate recover/3(start_in)
  s-p/1(data_out) -> NR LDPC Decoder/1  "ldpc_in"
  Sample Control Bus Selector1/1 -> p-p/2(start_in)
  Sample Control Bus Selector1/3 -> p-p/3(valid)
  rate recover/4(valid_out) -> s-p/2(valid_in)  "rm_out_valid"
  Constant3/1 -> NR LDPC Decoder/4
  Constant2/1 -> NR LDPC Decoder/3
  deinterleave/2(valid_out) -> rate recover/2(valid_in), Detect Rise Positive/1  "deinterleave_valid"
  synchronization/1(port1_syn) -> Delay2/1
  synchronization/2(port2_syn) -> Delay1/1
  port2_ctrl/1 -> synchronization/4(port2_ctrl)
  rxSig_tt1/1 -> synchronization/2(rxSig_tt)
  port1_ctrl/1 -> synchronization/3(port1_ctrl)
  chan_est_tt1/1 -> synchronization/1(chan_est_tt)
  synchronization/3(valid_syn) -> Detect Rise Positive1/1
  Detect Rise Positive1/1 -> synchronize_valid/1(start)
  Delay2/1 -> MRC/1(chan_est_tt)  "port1"
  Delay1/1 -> MRC/2(rxSig_tt)  "port2"
  synchronize_valid/1(valid_out) -> MRC/3(valid_tt)  "synchronize_valid"
  nVar_tt/1 -> soft demodule/1(nVar_tt)
  MRC/1(G_k_1) -> soft demodule/2(G_k_1)  "G_k_1"
  MRC/2(r_k) -> soft demodule/3(r_k)  "r_k"
  MRC/4(valid) -> soft demodule/5(valid)
  soft demodule/1(demod) -> deinterleave/1(data_tt)  "demod"
  soft demodule/2(valid_out) -> deinterleave/2(valid_tt)  "valid_in"
  MRC/3(start) -> soft demodule/4(start)
  NR CRC Decoder/1 -> data_out/1  "final_data"
  NR CRC Decoder/2 -> valid_out/1  "final_ctrl"

== system rx2/process10/OFDM_DEMOD1 ==
  process : Inport
  process_ctrl : Inport  Port=2  OutDataTypeStr=Bus: BUSOFDM1
  Bus Creator : BusCreator  Inputs=8
  Bus Selector : BusSelector  OutputSignals=signal11 (signal 1).valid,signal11 (signal 2).valid,signal11 (signal 3).valid,signal11 (signal 4).valid,signal11 (signal 5).valid,signal11 (signal 6).valid,signal11 (signal 7).valid,signal11 (signal 8).valid
  Demux : Demux  Outputs=8
  Mux : Mux  Inputs=8
  OFDM_demod1 : Subsystem
  OFDM_demod2 : Subsystem
  OFDM_demod3 : Subsystem
  OFDM_demod4 : Subsystem
  OFDM_demod5 : Subsystem
  OFDM_demod6 : Subsystem
  OFDM_demod7 : Subsystem
  OFDM_demod8 : Subsystem
  rxsig : Outport
  Rcrtl_out : Outport  Port=2  OutDataTypeStr=Bus: BUSOFDM1
  wires:
  Bus Creator/1 -> Rcrtl_out/1
  Mux/1 -> rxsig/1
  OFDM_demod7/1(data_out) -> Mux/8
  OFDM_demod4/1(data_out) -> Mux/4
  OFDM_demod1/2(ctrl_out) -> Bus Creator/1  "OFDM_ctrl_bf1_process1"
  OFDM_demod4/2(ctrl_out) -> Bus Creator/4  "OFDM_ctrl_bf1_process4"
  OFDM_demod6/1(data_out) -> Mux/6
  OFDM_demod8/1(data_out) -> Mux/7
  OFDM_demod6/2(ctrl_out) -> Bus Creator/6  "OFDM_ctrl_bf1_process6"
  OFDM_demod2/2(ctrl_out) -> Bus Creator/2  "OFDM_ctrl_bf1_process2"
  OFDM_demod1/1(data_out) -> Mux/1
  OFDM_demod5/1(data_out) -> Mux/5
  OFDM_demod8/2(ctrl_out) -> Bus Creator/7  "OFDM_ctrl_bf1_process7"
  OFDM_demod3/2(ctrl_out) -> Bus Creator/3  "OFDM_ctrl_bf1_process3"
  OFDM_demod3/1(data_out) -> Mux/3
  OFDM_demod7/2(ctrl_out) -> Bus Creator/8  "OFDM_ctrl_bf1_process8"
  OFDM_demod2/1(data_out) -> Mux/2
  OFDM_demod5/2(ctrl_out) -> Bus Creator/5  "OFDM_ctrl_bf1_process5"
  Bus Selector/1 -> OFDM_demod1/2(valid_in)  "<valid>"
  Demux/8 -> OFDM_demod7/1(ofdm_sym)
  Demux/7 -> OFDM_demod8/1(ofdm_sym)
  Demux/6 -> OFDM_demod6/1(ofdm_sym)
  Demux/5 -> OFDM_demod5/1(ofdm_sym)
  Bus Selector/8 -> OFDM_demod7/2(valid_in)  "<valid>"
  Bus Selector/7 -> OFDM_demod8/2(valid_in)  "<valid>"
  Bus Selector/6 -> OFDM_demod6/2(valid_in)  "<valid>"
  Bus Selector/5 -> OFDM_demod5/2(valid_in)  "<valid>"
  Bus Selector/4 -> OFDM_demod4/2(valid_in)  "<valid>"
  Demux/4 -> OFDM_demod4/1(ofdm_sym)
  Bus Selector/3 -> OFDM_demod3/2(valid_in)  "<valid>"
  Demux/3 -> OFDM_demod3/1(ofdm_sym)
  Bus Selector/2 -> OFDM_demod2/2(valid_in)  "<valid>"
  Demux/2 -> OFDM_demod2/1(ofdm_sym)
  Demux/1 -> OFDM_demod1/1(ofdm_sym)
  process/1 -> Demux/1
  process_ctrl/1 -> Bus Selector/1

== system rx2/process10/decoder ==
  chan_est_tt1 : Inport
  port1_ctrl : Inport  Port=2  OutDataTypeStr=Bus: BUSOFDM1
  rxSig_tt1 : Inport  Port=3
  port2_ctrl : Inport  Port=4  OutDataTypeStr=Bus: BUSOFDM1
  nVar_tt : Inport  Port=5  OutDataTypeStr=fixdt(0,16,12)
  Constant2 : Constant  OutDataTypeStr=boolean
  Constant3 : Constant  Value=72  OutDataTypeStr=uint16
  Delay1 : Delay  InitialCondition=0
  Delay2 : Delay  InitialCondition=0
  Detect Rise Positive : hdlsllib/Logic and Bit Operations/Detect Rise Positive  vinit=0  OutDataTypeStr=boolean
  Detect Rise Positive1 : hdlsllib/Logic and Bit Operations/Detect Rise Positive  vinit=0  OutDataTypeStr=boolean
  MRC : Subsystem
  NR CRC Decoder : whdledac/NR CRC Decoder  CRCType=CRC16  FullCheckSum=on  EnableCRCMaskPort=off  SimulateUsing=Code generation
  NR LDPC Decoder : whdledac/NR LDPC Decoder  Algorithm=Min-sum  ScalingFactor=0.75  Termination=Max  SpecifyInputs=Property  NumIterations=15  MaxNumIterations=30  RateCompatible=off  ParityCheckStatus=off  SimulateUsing=Code generation
  Sample Control Bus Selector1 : whdlutilities/Sample Control Bus Selector  OutputSignals=start,end,valid
  deinterleave : Subsystem  mask{length=1584}
      mask prompts: length "the length of data_in"
      mask DialogControl ParameterGroupVar Prompt: 参数
      mask DialogControl Control2 Prompt: the lantency is (length/2+3)
  p-p : Subsystem
  rate recover : Subsystem
  s-p : Subsystem
  soft demodule : Subsystem  mask{demod_length=1584}
      mask prompts: demod_length "The length of demod"
      mask DialogControl ParameterGroupVar Prompt: 参数
      mask DialogControl Control2 Prompt: Latency=4
  synchronization : Subsystem
  synchronize_valid : Subsystem  mask{valid_length=792}
      mask prompts: valid_length "The length of valid"
      mask DialogControl Control2 Prompt: Latency=2
  data_out : Outport
  valid_out : Outport  Port=2
  wires:
  NR CRC Decoder/2 -> valid_out/1  "final_ctrl"
  NR CRC Decoder/1 -> data_out/1  "final_data"
  MRC/3(start) -> soft demodule/4(start)
  soft demodule/2(valid_out) -> deinterleave/2(valid_tt)  "valid_in"
  soft demodule/1(demod) -> deinterleave/1(data_tt)  "demod"
  MRC/4(valid) -> soft demodule/5(valid)
  MRC/2(r_k) -> soft demodule/3(r_k)  "r_k"
  MRC/1(G_k_1) -> soft demodule/2(G_k_1)  "G_k_1"
  nVar_tt/1 -> soft demodule/1(nVar_tt)
  synchronize_valid/1(valid_out) -> MRC/3(valid_tt)  "synchronize_valid"
  Delay1/1 -> MRC/2(rxSig_tt)  "port2"
  Delay2/1 -> MRC/1(chan_est_tt)  "port1"
  Detect Rise Positive1/1 -> synchronize_valid/1(start)
  synchronization/3(valid_syn) -> Detect Rise Positive1/1
  chan_est_tt1/1 -> synchronization/1(chan_est_tt)
  port1_ctrl/1 -> synchronization/3(port1_ctrl)
  rxSig_tt1/1 -> synchronization/2(rxSig_tt)
  port2_ctrl/1 -> synchronization/4(port2_ctrl)
  synchronization/2(port2_syn) -> Delay1/1
  synchronization/1(port1_syn) -> Delay2/1
  deinterleave/2(valid_out) -> Detect Rise Positive/1, rate recover/2(valid_in)  "deinterleave_valid"
  Constant2/1 -> NR LDPC Decoder/3
  Constant3/1 -> NR LDPC Decoder/4
  rate recover/4(valid_out) -> s-p/2(valid_in)  "rm_out_valid"
  Sample Control Bus Selector1/3 -> p-p/3(valid)
  Sample Control Bus Selector1/1 -> p-p/2(start_in)
  s-p/1(data_out) -> NR LDPC Decoder/1  "ldpc_in"
  Detect Rise Positive/1 -> rate recover/3(start_in)
  rate recover/1(rate_recover) -> s-p/1(data_in)  "rm_out"
  NR LDPC Decoder/1 -> p-p/1(data_in)  "ldpc_out"
  NR LDPC Decoder/2 -> Sample Control Bus Selector1/1  "ldpc_out_ctrl"
  deinterleave/1(data_out) -> rate recover/1(demod)  "deinterleave_data"
  p-p/2(ctrl) -> NR CRC Decoder/2  "crc_in_ctrl"
  p-p/1(data) -> NR CRC Decoder/1  "crc_in"
  s-p/2(ctrl_out) -> NR LDPC Decoder/2  "ldpc_in_ctrl"
